simulink model "AccTarSel"  (R2018b)
settings: Solver=FixedStepDiscrete  StartTime=0.0  StopTime=inf  FixedStep=0.01  RelTol=1e-3
PostLoadFcn:
  | if any(exist('dsrtsu_mdlpostloadfcn', 'file') ~= 0), dsrtsu_mdlpostloadfcn('Execute', bdroot); end
values from neighbouring files (symbols this model uses):
  P_adtMaxBDC = 1.0    [AccTarSel.sldd]
  P_aFOCApproachIntpAcitve = -0.6    [AccTarSel.sldd]
  P_aFOCApproachIntpEnsure = -1.8    [AccTarSel.sldd]
  P_CutInEnable = 1.0    [AccTarSel.sldd]
  P_dAimMin = 4.5    [AccTarSel.sldd]
  P_dAimMinAVP = 1.5    [AccTarSel.sldd]
  P_dObjDrvOffMax = 5.0    [AccTarSel.sldd]
  P_dObjDrvOffMin = 3.0    [AccTarSel.sldd]
  P_dObjLowHystDecToStop = 4.5    [AccTarSel.sldd]
  P_dObjLowHystDecToStopAVP = 1.5    [AccTarSel.sldd]
  P_dObjUpperHystDecToStop = 5.0    [AccTarSel.sldd]
  P_dResMax = 5.0    [AccTarSel.sldd]
  P_dStandStill = 3.0    [AccTarSel.sldd]
  P_dStandStillMin = 2.0    [AccTarSel.sldd]
  P_dvarYMax4PO = 1.0    [AccTarSel.sldd]
  P_dyCutInThres = 3.6    [AccTarSel.sldd]
  P_facBDCInit = 0.7    [AccTarSel.sldd]
  P_facBDCIterCalc = 0.8    [AccTarSel.sldd]
  P_facFOCNegDiff = 0.3    [AccTarSel.sldd]
  P_facFOCPosDiff = 0.2    [AccTarSel.sldd]
  P_kapHystThres = 0.0005    [AccTarSel.sldd]
  P_PlausIntegDisable = 0.0    [AccTarSel.sldd]
  P_plausMin4PO = 0.5    [AccTarSel.sldd]
  P_probExistMin4PO = 0.8    [AccTarSel.sldd]
  P_StandObjEnable = 0.0    [AccTarSel.sldd]
  P_tAxTrackNegLower = 0.3    [AccTarSel.sldd]
  P_tAxTrackNegUpper = 0.6    [AccTarSel.sldd]
  P_tAxTrackPosLower = 1.0    [AccTarSel.sldd]
  P_tAxTrackPosUpper = 2.0    [AccTarSel.sldd]
  P_tBDCStartFilt = 0.2    [AccTarSel.sldd]
  P_tCSC = 3.5    [AccTarSel.sldd]
  P_tCurvFilt = 0.2    [AccTarSel.sldd]
  P_tCutInFilt = 0.5    [AccTarSel.sldd]
  P_tFiltAxAbsPONegFast = 0.1    [AccTarSel.sldd]
  P_tFiltAxAbsPONegSlow = 0.4    [AccTarSel.sldd]
  P_tFiltAxAbsPOPosFast = 1.2    [AccTarSel.sldd]
  P_tFiltAxAbsPOPosSlow = 2.0    [AccTarSel.sldd]
  P_tFiltAxAbsPOStand = 2.0    [AccTarSel.sldd]
  P_tFiltDAim = 0.1    [AccTarSel.sldd]
  P_tFiltDsd = 0.1    [AccTarSel.sldd]
  P_tFiltSpdLim = 3.0    [AccTarSel.sldd]
  P_tFiltVxAxPOFast = 0.15    [AccTarSel.sldd]
  P_tFiltVxAxPOSlow = 0.25    [AccTarSel.sldd]
  P_tFOCStatAccelFast = 4.0    [AccTarSel.sldd]
  P_tFOCStatAccelSlow = 3.5    [AccTarSel.sldd]
  P_tFOCStatDecelFast = 4.0    [AccTarSel.sldd]
  P_tFOCStatDecelSlow = 3.2    [AccTarSel.sldd]
  P_tMinDrvPhase = 2.0    [AccTarSel.sldd]
  P_tPredObjLeav = 1.2    [AccTarSel.sldd]
  P_tRollingFilt = 0.5    [AccTarSel.sldd]
  P_tRollingFinFilt = 1.0    [AccTarSel.sldd]
  P_tSSCNeg = 4.5    [AccTarSel.sldd]
  P_tSSCPos = 5.5    [AccTarSel.sldd]
  P_tToStop = 5.0    [AccTarSel.sldd]
  P_tToStopInBDC = 6.0    [AccTarSel.sldd]
  P_tToStopTrig = 4.0    [AccTarSel.sldd]
  P_vEgoDecToStop = 3.0    [AccTarSel.sldd]
  P_vEgoLowBDC = 4.0    [AccTarSel.sldd]
  P_vFOCNegDiff = 4.0    [AccTarSel.sldd]
  P_vFOCPosDiff = 5.0    [AccTarSel.sldd]
  P_vFOCStationaryFast = 15.0    [AccTarSel.sldd]
  P_vFOCStationarySlow = 5.0    [AccTarSel.sldd]
  P_vObjDrvOff = 0.5    [AccTarSel.sldd]
  P_vObjLowHystDecToStop = 0.5    [AccTarSel.sldd]
  P_vObjNoStop = 1.0    [AccTarSel.sldd]
  P_vObjReCalc = 1.0    [AccTarSel.sldd]
  P_vObjStop = 0.3    [AccTarSel.sldd]
  P_vObjUpperHystDecToStop = 0.8    [AccTarSel.sldd]
  P_vStandStill = 0.3    [AccTarSel.sldd]
  P_vStandStillHyst = 0.3    [AccTarSel.sldd]
  P_vyCutInThres = 0.5    [AccTarSel.sldd]
libraries: simulink x21, LPFilter x12
(part 6 of 11)

== system AccTarSel/ObjAdapter/For Each Subsystem/calcHist ==
  <trackStatus> : Inport
  Constant11 : Constant  Value=0  OutDataTypeStr=single
  Relational Operator : RelationalOperator  Operator=~=  OutDataTypeStr=boolean  RndMeth=Simplest
  Hist : Outport
  wires:
  Constant11/1 -> Relational Operator/1
  Relational Operator/1 -> Hist/1  "Hist"
  <trackStatus>/1 -> Relational Operator/2

== system AccTarSel/ObjRadarAdapter/For Each Subsystem/calcDx ==
  note: mass center
  note: rear axls to front bumper
  <longPosition> : Inport
  Add : Sum  Inputs=+-
  Constant1 : Constant  Value=3.68  OutDataTypeStr=single
  dx : Outport
  wires:
  <longPosition>/1 -> Add/1
  Constant1/1 -> Add/2
  Add/1 -> dx/1

== system AccTarSel/ObjRadarAdapter/For Each Subsystem/calcMotionSts ==
  note: Type:
      | 0	Unknown
      | 1	Pedestrain
      | 2	Bi/Motor cycle
      | >=3	Vehicle
  note: MotionSts:
      | 0	Unknown
      | 1	Standstill
      | 2	Driving
      | 3	InvDriving
      | 4	Stopped
      | 5	InvStopped
  MotionPattern : Inport
  1-D Lookup Table : Lookup_n-D  NumberOfTableDimensions=1  LookupTableObject=''  BreakpointsForDimension1=[0,1,2,3,4,5]  BreakpointsForDimension1FirstPoint=10  BreakpointsForDimension2FirstPoint=10  BreakpointsForDimension1Spacing=12  BreakpointsForDimension2Spacing=12  IndexSearchMethod=Linear search  Table=[0,1,4,2,2,0]  InterpMethod=Flat  InternalRulePriority=Speed  RndMeth=Simplest  InputSameDT=on
  MotionSts : Outport
  wires:
  MotionPattern/1 -> 1-D Lookup Table/1
  1-D Lookup Table/1 -> MotionSts/1

== system AccTarSel/ObjRadarAdapter/For Each Subsystem/calcType ==
  note: MotionSts:
      | 0	Unknown
      | 1	Standstill
      | 2	Driving
      | 3	InvDriving
      | 4	Stopped
      | 5	InvStopped
  note: Type:
      | 0	Unknown
      | 1	Pedestrain
      | 2	Bi/Motor cycle
      | >=3	Vehicle
  ObjType : Inport
  1-D Lookup Table : Lookup_n-D  NumberOfTableDimensions=1  LookupTableObject=''  BreakpointsForDimension1=[0,1,2,3]  BreakpointsForDimension1FirstPoint=10  BreakpointsForDimension2FirstPoint=10  BreakpointsForDimension1Spacing=12  BreakpointsForDimension2Spacing=12  IndexSearchMethod=Linear search  Table=[0,3,2,1]  InterpMethod=Flat  InternalRulePriority=Speed  RndMeth=Simplest  InputSameDT=on
  Type : Outport
  wires:
  1-D Lookup Table/1 -> Type/1
  ObjType/1 -> 1-D Lookup Table/1

== system AccTarSel/RTI Data/RTI Data Store/RTI Data Store ==
  RTI Data Store : Subsystem  mask(RTI_DATA_STORE){}
      mask help:
      | RTI Data Store Block. This block is used by RTI to store internal model dependent data. Deleting this block will result in data loss.
      |
      | NEVER DELETE, COPY, OR MODIFY THIS BLOCK!
      mask Help:
      | RTI Data Store Block. This block is used by RTI to store internal model dependent data. Deleting this block will result in data loss.
      | 
      | NEVER DELETE, COPY, OR MODIFY THIS BLOCK!
      mask Display: text(0.5, 0.5, ' ', 'HorizontalAlignment', 'center');

== system AccTarSel/Target_PreProcess/AVP_Target/If Action Subsystem ==
  note: Index = 200 -> AVP virtual target
  note: MotionSts:
      | 0	Unknown
      | 1	Standstill
      | 2	Driving
      | 3	InvDriving
      | 4	Stopped
      | 5	InvStopped
  note: Type:
      | 0	Unknown
      | 1	Pedestrain
      | 2	Bi/Motor cycle
      | >=3	Vehicle
      |
      | 20	AVP virtual target
  AVP_Info : Inport
  vRef : Inport  Port=2
  aRef : Inport  Port=3
  Action Port : ActionPort  ActionType=then
  Bus Creator2 : BusCreator  Inputs=11  OutDataTypeStr=Bus: ATS_PO_ST  NonVirtualBus=on
      settings: InheritFromInputs=off
  Bus Selector : BusSelector  OutputSignals=EndPoint_x
  Constant : Constant  OutDataTypeStr=boolean
  Constant1 : Constant  Value=200  OutDataTypeStr=single
  Constant10 : Constant  OutDataTypeStr=single
  Constant{3,5,7..8} (4 alike) : Constant  Value=0  OutDataTypeStr=single
  Constant9 : Constant  Value=20  OutDataTypeStr=single
  Gain : Gain  Gain=-1
  Gain1 : Gain  Gain=-1
  Virtual_Object : Outport
  wires:
  Constant8/1 -> Bus Creator2/9  "axAbs"
  Bus Selector/1 -> Bus Creator2/3  "<EndPoint_x>"
  Gain/1 -> Bus Creator2/5  "vx"
  Constant1/1 -> Bus Creator2/2  "Index"
  Constant5/1 -> Bus Creator2/6  "vy"
  aRef/1 -> Gain1/1
  Constant10/1 -> Bus Creator2/11  "MotionSts"
  Constant/1 -> Bus Creator2/1  "Valid"
  Constant7/1 -> Bus Creator2/8  "vxAbs"
  Constant3/1 -> Bus Creator2/4  "dy"
  Constant9/1 -> Bus Creator2/10  "Type"
  Bus Creator2/1 -> Virtual_Object/1
  vRef/1 -> Gain/1
  Gain1/1 -> Bus Creator2/7  "ax"
  AVP_Info/1 -> Bus Selector/1

== system AccTarSel/Target_PreProcess/AVP_Target/If Action Subsystem1 ==
  Action Port : ActionPort  ActionType=else
  Bus Creator2 : BusCreator  Inputs=11  OutDataTypeStr=Bus: ATS_PO_ST  NonVirtualBus=on
      settings: InheritFromInputs=off
  Constant : Constant  Value=0  OutDataTypeStr=boolean
  Constant1 : Constant  Value=255  OutDataTypeStr=single
  Constant{2..10} (9 alike) : Constant  Value=0  OutDataTypeStr=single
  Default : Outport
  wires:
  Constant/1 -> Bus Creator2/1  "Valid"
  Constant1/1 -> Bus Creator2/2  "Index"
  Constant2/1 -> Bus Creator2/3  "dx"
  Constant3/1 -> Bus Creator2/4  "dy"
  Constant4/1 -> Bus Creator2/5  "vx"
  Constant5/1 -> Bus Creator2/6  "vy"
  Constant6/1 -> Bus Creator2/7  "ax"
  Constant7/1 -> Bus Creator2/8  "vxAbs"
  Constant8/1 -> Bus Creator2/9  "axAbs"
  Constant9/1 -> Bus Creator2/10  "Type"
  Constant10/1 -> Bus Creator2/11  "MotionSts"
  Bus Creator2/1 -> Default/1

== system AccTarSel/Target_PreProcess/preFilt/Hold ==
  axTrackTime : Inport
  Action Port : ActionPort  ActionType=else
  Bus Selector : BusSelector  OutputSignals=NegTime,PosTime
  NegTime : Outport
  PosTime : Outport  Port=2
  wires:
  axTrackTime/1 -> Bus Selector/1
  Bus Selector/1 -> NegTime/1  "<NegTime>"
  Bus Selector/2 -> PosTime/1  "<PosTime>"

== system AccTarSel/Target_PreProcess/preFilt/NegTimeInc ==
  axTrackTime : Inport
  dT : Inport  Port=2
  Action Port : ActionPort  ActionType=then
  Add : Sum
  Bus Selector : BusSelector  OutputSignals=NegTime
  Constant : Constant  Value=5  OutDataTypeStr=single
  Constant1 : Constant  Value=0  OutDataTypeStr=single
  Max : MinMax  Inputs=2
  NegTime : Outport
  PosTime : Outport  Port=2
  wires:
  axTrackTime/1 -> Bus Selector/1
  Bus Selector/1 -> Add/2  "<NegTime>"
  dT/1 -> Add/1
  Add/1 -> Max/2
  Constant/1 -> Max/1
  Max/1 -> NegTime/1
  Constant1/1 -> PosTime/1

== system AccTarSel/Target_PreProcess/preFilt/PosTimeInc ==
  axTrackTime : Inport
  dT : Inport  Port=2
  Action Port : ActionPort  ActionType=elseif
  Add : Sum
  Bus Selector : BusSelector  OutputSignals=PosTime
  Constant : Constant  Value=5  OutDataTypeStr=single
  Constant1 : Constant  Value=0  OutDataTypeStr=single
  Max : MinMax  Inputs=2
  NegTime : Outport
  PosTime : Outport  Port=2
  wires:
  axTrackTime/1 -> Bus Selector/1
  Constant/1 -> Max/1
  Add/1 -> Max/2
  dT/1 -> Add/1
  Bus Selector/1 -> Add/2  "<PosTime>"
  Max/1 -> PosTime/1
  Constant1/1 -> NegTime/1

== system AccTarSel/ACC_Control/ArbitraryMix/calcAFOC/For Iterator Subsystem ==
  numFOC : Inport
  FOCInfo : Inport  Port=2
  Assignment1 : Assignment  IndexMode=Zero-based  DiagnosticForDimensions=Warning  IndexOptions=Index vector (port)  Indices=1  OutputSizes=1
  Assignment2 : Assignment  IndexMode=Zero-based  DiagnosticForDimensions=Warning  IndexOptions=Index vector (port)  Indices=1  OutputSizes=1
  Bus Selector : BusSelector  OutputSignals=aFOC,DecToStop
  For Iterator : ForIterator  IterationSource=external  IterationLimit=2  IndexMode=Zero-based
  Selector2 : Selector  IndexMode=Zero-based  InputPortWidth=6  IndexOptions=Index vector (port)  Indices=[1 3]  OutputSizes=1
  Zero1 : Constant  Value=zeros(1,6)  OutDataTypeStr=single
  Zero2 : Constant  Value=zeros(1,6)  OutDataTypeStr=boolean
  aFOCArray : Outport
  DecToStopArray : Outport  Port=2
  wires:
  numFOC/1 -> For Iterator/1
  Zero1/1 -> Assignment1/1
  [i_cnt] -> Assignment1/3
  Assignment1/1 -> aFOCArray/1
  Bus Selector/1 -> Assignment1/2  "<aFOC>"
  FOCInfo/1 -> Selector2/1
  For Iterator/1 -> Selector2/2, [i_cnt]  "i_cnt"
  Selector2/1 -> Bus Selector/1
  Bus Selector/2 -> Assignment2/2  "<DecToStop>"
  [i_cnt] -> Assignment2/3
  Zero2/1 -> Assignment2/1
  Assignment2/1 -> DecToStopArray/1

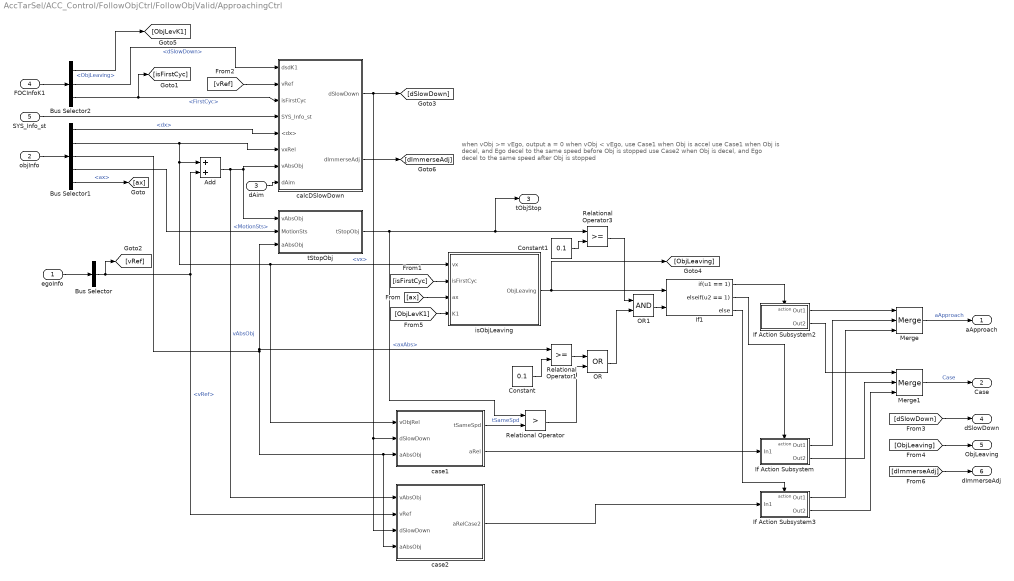
== system AccTarSel/ACC_Control/FollowObjCtrl/FollowObjValid/ApproachingCtrl ==
  note: when vObj >= vEgo, output a = 0
      | when vObj < vEgo, use Case1 when Obj is accel
      | 				  use Case1 when Obj is decel, and Ego decel to the same speed before Obj is stopped
      | 				  use Case2 when Obj is decel, and Ego decel to the same speed after Obj is stopped
  egoInfo : Inport
  objInfo : Inport  Port=2
  dAim : Inport  Port=3
  FOCInfoK1 : Inport  Port=4
  SYS_Info_st : Inport  Port=5
  Add : Sum
  Bus Selector : BusSelector  OutputSignals=vRef
  Bus Selector1 : BusSelector  OutputSignals=dx,vx,axAbs,MotionSts,ax
  Bus Selector2 : BusSelector  OutputSignals=ObjLeaving,dSlowDown,FirstCyc
  Constant : Constant  Value=0.1  OutDataTypeStr=single
  Constant1 : Constant  Value=0.1  OutDataTypeStr=single
  If Action Subsystem : Subsystem  TreatAsAtomicUnit=on
  If Action Subsystem2 : Subsystem  TreatAsAtomicUnit=on
  If Action Subsystem3 : Subsystem  TreatAsAtomicUnit=on
  If1 : If  NumInputs=2  IfExpression=u1 == 1  ElseIfExpressions=u2 == 1
  Merge : Merge  Inputs=3
  Merge1 : Merge  Inputs=3
  OR : Logic  Operator=OR  AllPortsSameDT=off  OutDataTypeStr=boolean
  OR1 : Logic  AllPortsSameDT=off  OutDataTypeStr=boolean
  Relational Operator : RelationalOperator  Operator=>  OutDataTypeStr=boolean  RndMeth=Simplest
  Relational Operator1 : RelationalOperator  OutDataTypeStr=boolean  RndMeth=Simplest
  Relational Operator3 : RelationalOperator  OutDataTypeStr=boolean  RndMeth=Simplest
  calcDSlowDown : Subsystem
  case1 : Subsystem
  case2 : Subsystem
  isObjLeaving : Subsystem
  tStopObj : Subsystem
  aApproach : Outport
  Case : Outport  Port=2
  tObjStop : Outport  Port=3
  dSlowDown : Outport  Port=4
  ObjLeaving : Outport  Port=5
  dImmerseAdj : Outport  Port=6
  wires:
  egoInfo/1 -> Bus Selector/1
  objInfo/1 -> Bus Selector1/1
  Add/1 -> tStopObj/1(vAbsObj), calcDSlowDown/7(vAbsObj), case2/1(vAbsObj)  "vAbsObj"
  Bus Selector/1 -> [vRef], case2/2(vRef), Add/2  "<vRef>"
  Bus Selector1/2 -> Add/1, case1/1(vObjRel), isObjLeaving/1(vx), calcDSlowDown/6(vxRel)  "<vx>"
  Bus Selector1/1 -> calcDSlowDown/5(<dx>)  "<dx>"
  If1/1 -> If Action Subsystem2/Action
  calcDSlowDown/1(dSlowDown) -> case2/3(dSlowDown), case1/2(dSlowDown), [dSlowDown]
  Bus Selector1/3 -> tStopObj/3(aAbsObj), Relational Operator1/1, case2/4(aAbsObj), case1/3(aAbsObj)  "<axAbs>"
  case1/2(aRel) -> If Action Subsystem/1(In1)
  If1/2 -> If Action Subsystem/Action
  tStopObj/1(tStopObj) -> tObjStop/1, Relational Operator3/1, Relational Operator/1
  Constant/1 -> Relational Operator1/2
  Relational Operator1/1 -> OR/1
  Relational Operator/1 -> OR/2
  case2/1(aRelCase2) -> If Action Subsystem3/1(In1)
  If Action Subsystem/1(Out1) -> Merge/2
  If Action Subsystem2/1(Out1) -> Merge/1
  If Action Subsystem3/1(Out1) -> Merge/3
  Merge/1 -> aApproach/1  "aApproach"
  isObjLeaving/1(ObjLeaving) -> [ObjLeaving], If1/1
  case1/1(tSameSpd) -> Relational Operator/2  "tSameSpd"
  Bus Selector1/4 -> tStopObj/2(MotionSts)  "<MotionSts>"
  If1/3 -> If Action Subsystem3/Action
  OR/1 -> OR1/2
  Relational Operator3/1 -> OR1/1
  OR1/1 -> If1/2
  Bus Selector2/3 -> [isFirstCyc], calcDSlowDown/3(isFirstCyc)  "<FirstCyc>"
  SYS_Info_st/1 -> calcDSlowDown/4(SYS_Info_st)
  dAim/1 -> calcDSlowDown/8(dAim)
  Bus Selector1/5 -> [ax]  "<ax>"
  Constant1/1 -> Relational Operator3/2
  [isFirstCyc] -> isObjLeaving/2(isFirstCyc)
  [ax] -> isObjLeaving/3(ax)
  If Action Subsystem2/2(Out2) -> Merge1/1
  If Action Subsystem/2(Out2) -> Merge1/2
  If Action Subsystem3/2(Out2) -> Merge1/3
  Merge1/1 -> Case/1  "Case"
  [vRef] -> calcDSlowDown/2(vRef)
  [dSlowDown] -> dSlowDown/1
  [ObjLeaving] -> ObjLeaving/1
  FOCInfoK1/1 -> Bus Selector2/1
  Bus Selector2/2 -> calcDSlowDown/1(dsdK1)  "<dSlowDown>"
  Bus Selector2/1 -> [ObjLevK1]  "<ObjLeaving>"
  [ObjLevK1] -> isObjLeaving/4(K1)
  calcDSlowDown/2(dImmerseAdj) -> [dImmerseAdj]
  [dImmerseAdj] -> dImmerseAdj/1

== system AccTarSel/ACC_Control/FollowObjCtrl/FollowObjValid/BrakeDistCtrl ==
  note: BDC_State
      | 0	PASSIVE
      | 1	CALC
      | 2	ACTIVE
      | 3	RECALC
  aCvK1 : Inport
  SYS_Info_st : Inport  Port=2
  egoInfo : Inport  Port=3
  objInfo : Inport  Port=4
  BDC_State_Machine : Stateflow chart  TreatAsAtomicUnit=on
  Bus Creator : BusCreator  Inputs=5
  Memory : Memory
  Memory1 : Memory
  Memory2 : Memory
  To Workspace : ToWorkspace  VariableName=simout  SaveFormat=Timeseries  SampleTime=-1
  calcA : Subsystem
  calcCriteria : Subsystem
  calcProfile : Subsystem
  BDC_Acitve : Outport
  aBDC : Outport  Port=2
  BDC_State : Outport  Port=3
  wires:
  egoInfo/1 -> calcProfile/1(egoInfo), calcCriteria/4(egoInfo)
  objInfo/1 -> calcProfile/4(objInfo), calcCriteria/5(objInfo)
  calcCriteria/3(egoLowSpd) -> BDC_State_Machine/3(egoLowSpd)
  calcCriteria/1(ObjToStop) -> BDC_State_Machine/1(ObjToStop)
  calcCriteria/2(ObjToStopTrig) -> BDC_State_Machine/2(ObjToStopTrig)
  calcCriteria/4(PreStop) -> BDC_State_Machine/4(PreStop)
  calcCriteria/5(ProfileReCalc) -> BDC_State_Machine/5(ProfileReCalc)
  BDC_State_Machine/1(BDC_State) -> Memory/1, calcProfile/2(BDC_State), calcA/1(State), Bus Creator/4, BDC_State/1  "BDC_State"
  calcCriteria/6(dObjToStop) -> calcProfile/3(dObjToStop)
  BDC_State_Machine/2(tElapse) -> Memory2/1, Bus Creator/3, calcA/3(tElapse)
  calcA/2(a_BDC) -> Bus Creator/5, aBDC/1  "aBDC"
  SYS_Info_st/1 -> calcA/5(SYS_Info_st), BDC_State_Machine/6(SYS_Info_st)
  Bus Creator/1 -> To Workspace/1
  Memory/1 -> calcCriteria/2(BDC_StateK1)
  calcProfile/1(Profile) -> Memory1/1, Bus Creator/2, calcA/2(Profile)
  Memory1/1 -> calcCriteria/3(ProfileK1)
  Memory2/1 -> calcCriteria/1(tElaps)
  calcCriteria/7(dRes) -> calcA/4(dRes)
  aCvK1/1 -> calcProfile/5(aCvK1)
  calcA/1(BDC_Acitve) -> BDC_Acitve/1

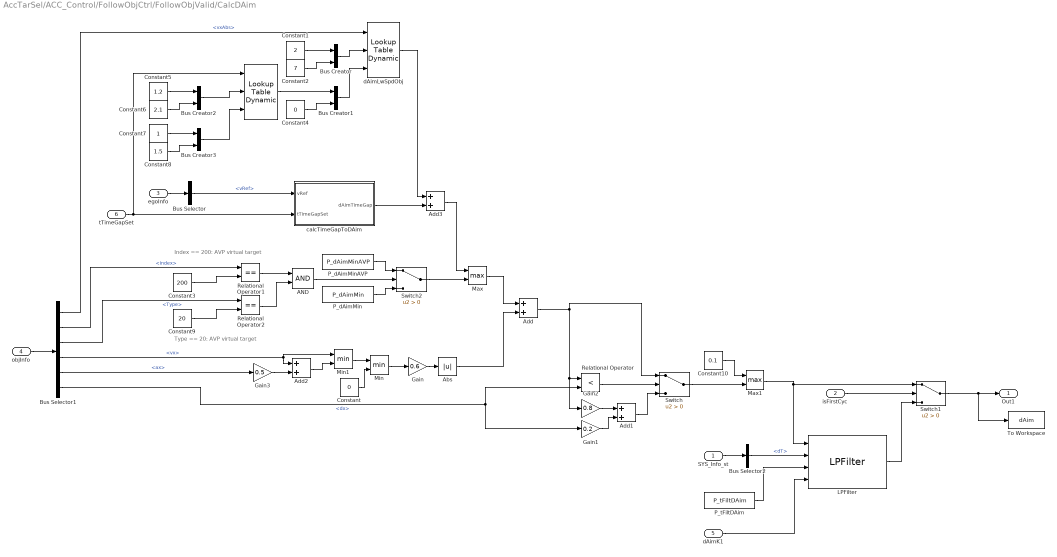
== system AccTarSel/ACC_Control/FollowObjCtrl/FollowObjValid/CalcDAim ==
  note: Index == 200: AVP virtual target
  note: Type == 20: AVP virtual target
  SYS_Info_st : Inport
  isFirstCyc : Inport  Port=2
  egoInfo : Inport  Port=3
  objInfo : Inport  Port=4
  dAimK1 : Inport  Port=5
  tTimeGapSet : Inport  Port=6
  " " : simulink/Lookup Tables/Lookup Table Dynamic  LookUpMeth=Interpolation-Use End Values  OutDataType=fixdt('single')  OutScaling=[]  OutputDataTypeScalingMode=Specify via dialog  OutDataTypeStr=single  DoSatur=off
      settings: SourceProductName=Simulink
  AND : Logic  AllPortsSameDT=off  OutDataTypeStr=boolean
  Abs : Abs
  Add{,1..3} (4 alike) : Sum
  Bus Creator{,1..3} (4 alike) : BusCreator  Inputs=2
  Bus Selector : BusSelector  OutputSignals=vRef
  Bus Selector1 : BusSelector  OutputSignals=vxAbs,Index,Type,vx,ax,dx
  Bus Selector2 : BusSelector  OutputSignals=dT
  Constant : Constant  Value=0  OutDataTypeStr=single
  Constant1 : Constant  Value=2  OutDataTypeStr=single
  Constant10 : Constant  Value=0.1  OutDataTypeStr=single
  Constant2 : Constant  Value=7  OutDataTypeStr=single
  Constant3 : Constant  Value=200  OutDataTypeStr=single
  Constant4 : Constant  Value=0  OutDataTypeStr=single
  Constant5 : Constant  Value=1.2  OutDataTypeStr=single
  Constant6 : Constant  Value=2.1  OutDataTypeStr=single
  Constant7 : Constant  OutDataTypeStr=single
  Constant8 : Constant  Value=1.5  OutDataTypeStr=single
  Constant9 : Constant  Value=20  OutDataTypeStr=single
  Gain : Gain  Gain=0.6
  Gain1 : Gain  Gain=0.2
  Gain2 : Gain  Gain=0.8
  Gain3 : Gain  Gain=0.5
  LPFilter : LPFilter/LPFilter  SystemSampleTime=-1
      settings: SourceProductName=CustomLib
  Max : MinMax  Function=max  Inputs=2
  Max1 : MinMax  Function=max  Inputs=2
  Min : MinMax  Inputs=2
  Min1 : MinMax  Inputs=2
  P_dAimMin : Constant  Value=P_dAimMin  OutDataTypeStr=single
  P_dAimMinAVP : Constant  Value=P_dAimMinAVP  OutDataTypeStr=single
  P_tFiltDAim : Constant  Value=P_tFiltDAim  OutDataTypeStr=single
  Relational Operator : RelationalOperator  Operator=<  OutDataTypeStr=boolean  RndMeth=Simplest
  Relational Operator1 : RelationalOperator  Operator===  OutDataTypeStr=boolean  RndMeth=Simplest
  Relational Operator2 : RelationalOperator  Operator===  OutDataTypeStr=boolean  RndMeth=Simplest
  Switch : Switch  Criteria=u2 > Threshold
  Switch1 : Switch  Criteria=u2 > Threshold
  Switch2 : Switch  Criteria=u2 > Threshold
  To Workspace : ToWorkspace  VariableName=dAim  SaveFormat=Timeseries  SampleTime=-1
  calcTimeGapToDAim : Subsystem
  dAimLwSpdObj : simulink/Lookup Tables/Lookup Table Dynamic  LookUpMeth=Interpolation-Use End Values  OutDataType=fixdt('single')  OutScaling=[]  OutputDataTypeScalingMode=Specify via dialog  OutDataTypeStr=single  DoSatur=off
      settings: SourceProductName=Simulink
  Out1 : Outport
  wires:
  egoInfo/1 -> Bus Selector/1
  tTimeGapSet/1 -> calcTimeGapToDAim/2(tTimeGapSet), " "/1
  Add/1 -> Switch/1, Gain2/1, Relational Operator/1
  objInfo/1 -> Bus Selector1/1
  Constant/1 -> Min/2
  Min/1 -> Gain/1
  Gain/1 -> Abs/1
  Abs/1 -> Add/2
  Bus Selector1/6 -> Relational Operator/2, Gain1/1  "<dx>"
  Relational Operator/1 -> Switch/2
  Gain2/1 -> Add1/1
  Gain1/1 -> Add1/2
  Add1/1 -> Switch/3
  isFirstCyc/1 -> Switch1/2
  Max1/1 -> LPFilter/1, Switch1/1
  SYS_Info_st/1 -> Bus Selector2/1
  Bus Selector2/1 -> LPFilter/2  "<dT>"
  dAimK1/1 -> LPFilter/4
  LPFilter/1 -> Switch1/3
  Switch1/1 -> To Workspace/1, Out1/1
  P_tFiltDAim/1 -> LPFilter/3
  Max/1 -> Add/1
  Bus Selector1/5 -> Gain3/1  "<ax>"
  Gain3/1 -> Add2/2
  Bus Selector1/4 -> Add2/1, Min1/1  "<vx>"
  Add2/1 -> Min1/2
  Min1/1 -> Min/1
  Bus Selector1/1 -> dAimLwSpdObj/1  "<vxAbs>"
  Constant4/1 -> Bus Creator1/2
  Bus Creator1/1 -> dAimLwSpdObj/3
  " "/1 -> Bus Creator1/1
  dAimLwSpdObj/1 -> Add3/1
  Constant2/1 -> Bus Creator/2
  Bus Creator/1 -> dAimLwSpdObj/2
  Constant1/1 -> Bus Creator/1
  calcTimeGapToDAim/1(dAimTimeGap) -> Add3/2
  Add3/1 -> Max/1
  Constant5/1 -> Bus Creator2/1
  Bus Creator2/1 -> " "/2
  Constant6/1 -> Bus Creator2/2
  Constant7/1 -> Bus Creator3/1
  Bus Creator3/1 -> " "/3
  Constant8/1 -> Bus Creator3/2
  Bus Selector/1 -> calcTimeGapToDAim/1(vRef)  "<vRef>"
  Bus Selector1/2 -> Relational Operator1/1  "<Index>"
  Constant3/1 -> Relational Operator1/2
  Bus Selector1/3 -> Relational Operator2/1  "<Type>"
  Constant9/1 -> Relational Operator2/2
  Relational Operator1/1 -> AND/1
  Relational Operator2/1 -> AND/2
  AND/1 -> Switch2/2
  P_dAimMinAVP/1 -> Switch2/1
  P_dAimMin/1 -> Switch2/3
  Switch2/1 -> Max/2
  Switch/1 -> Max1/2
  Constant10/1 -> Max1/1
